simulink library "ammclib_bam_s32k14x"  (Simulink 9.0)
settings: Solver=ode45  StartTime=0.0  StopTime=10.0  RelTol=1e-3
undefined symbols (not defined in the file): f16A1, f16A2, f16B0, f16B1, f16B2, f16C1, f16CC1, f16CC1sc, f16CC1sc_D, f16CC1sc_Q, f16CC1scD, f16CC1scQ, f16CC2, f16CC2sc, f16CC2sc_D, f16CC2sc_Q, f16CC2scD, f16CC2scQ, f16DerivGain, f16EGain, f16FiltCoef, f16HystOff, f16HystOn, f16IGain, f16IntegGain, f16IntegGainFW, f16IntegGainQ, f16Kd, f16Kq, f16Limit, f16LowerLim, f16LowerLimit_D, f16LowerLimit_Q, f16ModIndex, f16OutValOff, f16OutValOn, f16PropGain, f16PropGainFW, f16PropGainQ, f16RampDown, f16RampUp, f16UGain, f16UpperLim, f16UpperLimit, f16UpperLimit_D, f16UpperLimit_Q, f16WIGain, f32A1, f32A2, f32B0, f32B1, f32B2, f32C1, f32CC1, f32CC1sc, f32CC1sc_D, f32CC1sc_Q, f32CC1scD, f32CC1scQ, f32CC2 ... (+122)
(part 3 of 11)

== system ammclib_bam_s32k14x/GMCLIB/bam_f32 ==
  GMCLIB_ClarkInv_F32 : Subsystem  mask(GMCLIB_ClarkInv_F32){}
      mask help: Bit accurate model of inverse Clarke transformation 2ph -> 3ph
      mask init:
      | pos = get_param(gcb, 'Position');width = pos(3) - pos(1); height = pos(4) - pos(2);tX=width/2;tY=height*0.9;
      mask Help: web(fullfile(mbd_s32k_mc_block_help('s32k14x'), 'S32K14XMCLUG.pdf'), '-browser')
      mask Display: color('black');port_label('input',1,'f32Alpha');port_label('input',2,'f32Beta');port_label('output',1,'f32A');port_label('output',2,'f32B');port_label('output',3,'f32C');color('black');disp('GMCLIB_ClarkInv_F32');color('blue');text(tX,tY, 'BAM', 'horizontalAlignment', 'center');
  GMCLIB_Clark_F32 : Subsystem  mask(GMCLIB_Clark_F32){}
      mask help: Bit accurate model of Clarke transformation 3ph -> 2ph.
      mask init:
      | pos = get_param(gcb, 'Position');width = pos(3) - pos(1); height = pos(4) - pos(2);tX=width/2;tY=height*0.9;
      mask Help: web(fullfile(mbd_s32k_mc_block_help('s32k14x'), 'S32K14XMCLUG.pdf'), '-browser')
      mask Display: color('black');port_label('input',1,'f32A');port_label('input',2,'f32B');port_label('input',3,'f32C');port_label('output',1,'f32Alpha');port_label('output',2,'f32Beta');color('black');disp('GMCLIB_Clark_F32');color('blue');text(tX,tY, 'BAM', 'horizontalAlignment', 'center');
  GMCLIB_DecouplingPMSM_F32 : Subsystem  mask(GMCLIB_DecouplingPMSM_F32){f32Kd=f32Kd, s16KdShift=s16KdShift, f32Kq=f32Kq, s16KqShift=s16KqShift}
      mask help: Bit accurate model of decoupling for PMSM model.
      mask init:
      | pos = get_param(gcb, 'Position');width = pos(3) - pos(1); height = pos(4) - pos(2);tX=width/2;tY=height*0.9;
      mask Help: web(fullfile(mbd_s32k_mc_block_help('s32k14x'), 'S32K14XMCLUG.pdf'), '-browser')
      mask Display: color('black');port_label('input',1,'f32Ud');port_label('input',2,'f32Uq');port_label('input',3,'f32Id');port_label('input',4,'f32Iq');port_label('input',5,'f32AngVel');port_label('output',1,'f32UdDec');port_label('output',2,'f32UqDec');color('black');disp('GMCLIB_DecouplingPMSM_F32');color('blue');text(tX,tY, 'BAM', 'horizontalAlignment', 'center');
  GMCLIB_ElimDcBusRip_F32 : Subsystem  mask(GMCLIB_ElimDcBusRip_F32){f32ModIndex=f32ModIndex}
      mask help: Bit accurate model of DC Bus voltage ripple elimination function.
      mask init:
      | pos = get_param(gcb, 'Position');width = pos(3) - pos(1); height = pos(4) - pos(2);tX=width/2;tY=height*0.9;
      mask Help: web(fullfile(mbd_s32k_mc_block_help('s32k14x'), 'S32K14XMCLUG.pdf'), '-browser')
      mask Display: color('black');port_label('input',1,'f32Alpha');port_label('input',2,'f32Beta');port_label('input',3,'f32ArgDcBusMsr');port_label('output',1,'f32AlphaOut');port_label('output',2,'f32BetaOut');color('black');disp('GMCLIB_ElimDcBusRip_F32');color('blue');text(tX,tY, 'BAM', 'horizontalAlignment', 'center');
  GMCLIB_ParkInv_F32 : Subsystem  mask(GMCLIB_ParkInv_F32){}
      mask help: Bit accurate model of Inverse Park transformation 2ph rotational -> 2ph stationary.
      mask init:
      | pos = get_param(gcb, 'Position');width = pos(3) - pos(1); height = pos(4) - pos(2);tX=width/2;tY=height*0.9;
      mask Help: web(fullfile(mbd_s32k_mc_block_help('s32k14x'), 'S32K14XMCLUG.pdf'), '-browser')
      mask Display: color('black');port_label('input',1,'f32D');port_label('input',2,'f32Q');port_label('input',3,'f32Sin');port_label('input',4,'f32Cos');port_label('output',1,'f32Alpha');port_label('output',2,'f32Beta');color('black');disp('GMCLIB_ParkInv_F32');color('blue');text(tX,tY, 'BAM', 'horizontalAlignment', 'center');
  GMCLIB_Park_F32 : Subsystem  mask(GMCLIB_Park_F32){}
      mask help: Bit accurate model of Park transformation 2ph stationary -> 2ph rotational.
      mask init:
      | pos = get_param(gcb, 'Position');width = pos(3) - pos(1); height = pos(4) - pos(2);tX=width/2;tY=height*0.9;
      mask Help: web(fullfile(mbd_s32k_mc_block_help('s32k14x'), 'S32K14XMCLUG.pdf'), '-browser')
      mask Display: color('black');port_label('input',1,'f32Alpha');port_label('input',2,'f32Beta');port_label('input',3,'f32Sin');port_label('input',4,'f32Cos');port_label('output',1,'f32D');port_label('output',2,'f32Q');color('black');disp('GMCLIB_Park_F32');color('blue');text(tX,tY, 'BAM', 'horizontalAlignment', 'center');
  GMCLIB_PwmIct_F32 : Subsystem  mask(GMCLIB_PwmIct_F32){}
      mask help: Bit accurate model of General Sinusoidal PWM.
      mask init:
      | pos = get_param(gcb, 'Position');width = pos(3) - pos(1); height = pos(4) - pos(2);tX=width/2;tY=height*0.9;
      mask Help: web(fullfile(mbd_s32k_mc_block_help('s32k14x'), 'S32K14XMCLUG.pdf'), '-browser')
      mask Display: color('black');port_label('input',1,'f32In1');port_label('input',2,'f32In2');port_label('output',1,'f32Out1');port_label('output',2,'f32Out2');port_label('output',3,'f32Out3');port_label('output',4,'u32Sector');color('black');disp('GMCLIB_PwmIct_F32');color('blue');text(tX,tY, 'BAM', 'horizontalAlignment', 'center');
  GMCLIB_SvmStd_F32 : Subsystem  mask(GMCLIB_SvmStd_F32){}
      mask help: Bit accurate model of Standard Space Vector Modulation.
      mask init:
      | pos = get_param(gcb, 'Position');width = pos(3) - pos(1); height = pos(4) - pos(2);tX=width/2;tY=height*0.9;
      mask Help: web(fullfile(mbd_s32k_mc_block_help('s32k14x'), 'S32K14XMCLUG.pdf'), '-browser')
      mask Display: color('black');port_label('input',1,'f32In1');port_label('input',2,'f32In2');port_label('output',1,'f32Out1');port_label('output',2,'f32Out2');port_label('output',3,'f32Out3');port_label('output',4,'u32Sector');color('black');disp('GMCLIB_SvmStd_F32');color('blue');text(tX,tY, 'BAM', 'horizontalAlignment', 'center');
  GMCLIB_SvmU0n_F32 : Subsystem  mask(GMCLIB_SvmU0n_F32){}
      mask help: Bit accurate model of Standard Space Vector Modulation.
      mask init:
      | pos = get_param(gcb, 'Position');width = pos(3) - pos(1); height = pos(4) - pos(2);tX=width/2;tY=height*0.9;
      mask Help: web(fullfile(mbd_s32k_mc_block_help('s32k14x'), 'S32K14XMCLUG.pdf'), '-browser')
      mask Display: color('black');port_label('input',1,'f32In1');port_label('input',2,'f32In2');port_label('output',1,'f32Out1');port_label('output',2,'f32Out2');port_label('output',3,'f32Out3');port_label('output',4,'u32Sector');color('black');disp('GMCLIB_SvmU0n_F32');color('blue');text(tX,tY, 'BAM', 'horizontalAlignment', 'center');

== system ammclib_bam_s32k14x/GMCLIB/bam_flt ==
  GMCLIB_ClarkInv_FLT : Subsystem  mask(GMCLIB_ClarkInv_FLT){}
      mask help: Bit accurate model of inverse Clarke transformation 2ph -> 3ph
      mask init:
      | pos = get_param(gcb, 'Position');width = pos(3) - pos(1); height = pos(4) - pos(2);tX=width/2;tY=height*0.9;
      mask Help: web(fullfile(mbd_s32k_mc_block_help('s32k14x'), 'S32K14XMCLUG.pdf'), '-browser')
      mask Display: color('black');port_label('input',1,'fltAlpha');port_label('input',2,'fltBeta');port_label('output',1,'fltA');port_label('output',2,'fltB');port_label('output',3,'fltC');color('black');disp('GMCLIB_ClarkInv_FLT');color('blue');text(tX,tY, 'BAM', 'horizontalAlignment', 'center');
  GMCLIB_Clark_FLT : Subsystem  mask(GMCLIB_Clark_FLT){}
      mask help: Bit accurate model of Clarke transformation 3ph -> 2ph.
      mask init:
      | pos = get_param(gcb, 'Position');width = pos(3) - pos(1); height = pos(4) - pos(2);tX=width/2;tY=height*0.9;
      mask Help: web(fullfile(mbd_s32k_mc_block_help('s32k14x'), 'S32K14XMCLUG.pdf'), '-browser')
      mask Display: color('black');port_label('input',1,'fltA');port_label('input',2,'fltB');port_label('input',3,'fltC');port_label('output',1,'fltAlpha');port_label('output',2,'fltBeta');color('black');disp('GMCLIB_Clark_FLT');color('blue');text(tX,tY, 'BAM', 'horizontalAlignment', 'center');
  GMCLIB_DecouplingPMSM_FLT : Subsystem  mask(GMCLIB_DecouplingPMSM_FLT){fltKd=fltKd, fltKq=fltKq}
      mask help: Bit accurate model of decoupling for PMSM model.
      mask init:
      | pos = get_param(gcb, 'Position');width = pos(3) - pos(1); height = pos(4) - pos(2);tX=width/2;tY=height*0.9;
      mask Help: web(fullfile(mbd_s32k_mc_block_help('s32k14x'), 'S32K14XMCLUG.pdf'), '-browser')
      mask Display: color('black');port_label('input',1,'fltUd');port_label('input',2,'fltUq');port_label('input',3,'fltId');port_label('input',4,'fltIq');port_label('input',5,'fltAngVel');port_label('output',1,'fltUdDec');port_label('output',2,'fltUqDec');color('black');disp('GMCLIB_DecouplingPMSM_FLT');color('blue');text(tX,tY, 'BAM', 'horizontalAlignment', 'center');
  GMCLIB_ElimDcBusRip_FLT : Subsystem  mask(GMCLIB_ElimDcBusRip_FLT){fltModIndex=fltModIndex}
      mask help: Bit accurate model of DC Bus voltage ripple elimination function.
      mask init:
      | pos = get_param(gcb, 'Position');width = pos(3) - pos(1); height = pos(4) - pos(2);tX=width/2;tY=height*0.9;
      mask Help: web(fullfile(mbd_s32k_mc_block_help('s32k14x'), 'S32K14XMCLUG.pdf'), '-browser')
      mask Display: color('black');port_label('input',1,'fltAlpha');port_label('input',2,'fltBeta');port_label('input',3,'fltArgDcBusMsr');port_label('output',1,'fltAlphaOut');port_label('output',2,'fltBetaOut');color('black');disp('GMCLIB_ElimDcBusRip_FLT');color('blue');text(tX,tY, 'BAM', 'horizontalAlignment', 'center');
  GMCLIB_ParkInv_FLT : Subsystem  mask(GMCLIB_ParkInv_FLT){}
      mask help: Bit accurate model of Inverse Park transformation 2ph rotational -> 2ph stationary.
      mask init:
      | pos = get_param(gcb, 'Position');width = pos(3) - pos(1); height = pos(4) - pos(2);tX=width/2;tY=height*0.9;
      mask Help: web(fullfile(mbd_s32k_mc_block_help('s32k14x'), 'S32K14XMCLUG.pdf'), '-browser')
      mask Display: color('black');port_label('input',1,'fltD');port_label('input',2,'fltQ');port_label('input',3,'fltSin');port_label('input',4,'fltCos');port_label('output',1,'fltAlpha');port_label('output',2,'fltBeta');color('black');disp('GMCLIB_ParkInv_FLT');color('blue');text(tX,tY, 'BAM', 'horizontalAlignment', 'center');
  GMCLIB_Park_FLT : Subsystem  mask(GMCLIB_Park_FLT){}
      mask help: Bit accurate model of Park transformation 2ph stationary -> 2ph rotational.
      mask init:
      | pos = get_param(gcb, 'Position');width = pos(3) - pos(1); height = pos(4) - pos(2);tX=width/2;tY=height*0.9;
      mask Help: web(fullfile(mbd_s32k_mc_block_help('s32k14x'), 'S32K14XMCLUG.pdf'), '-browser')
      mask Display: color('black');port_label('input',1,'fltAlpha');port_label('input',2,'fltBeta');port_label('input',3,'fltSin');port_label('input',4,'fltCos');port_label('output',1,'fltD');port_label('output',2,'fltQ');color('black');disp('GMCLIB_Park_FLT');color('blue');text(tX,tY, 'BAM', 'horizontalAlignment', 'center');
  GMCLIB_PwmIct_FLT : Subsystem  mask(GMCLIB_PwmIct_FLT){}
      mask help: Bit accurate model of General Sinusoidal PWM.
      mask init:
      | pos = get_param(gcb, 'Position');width = pos(3) - pos(1); height = pos(4) - pos(2);tX=width/2;tY=height*0.9;
      mask Help: web(fullfile(mbd_s32k_mc_block_help('s32k14x'), 'S32K14XMCLUG.pdf'), '-browser')
      mask Display: color('black');port_label('input',1,'fltIn1');port_label('input',2,'fltIn2');port_label('output',1,'fltOut1');port_label('output',2,'fltOut2');port_label('output',3,'fltOut3');port_label('output',4,'u32Sector');color('black');disp('GMCLIB_PwmIct_FLT');color('blue');text(tX,tY, 'BAM', 'horizontalAlignment', 'center');
  GMCLIB_SvmStd_FLT : Subsystem  mask(GMCLIB_SvmStd_FLT){}
      mask help: Bit accurate model of Standard Space Vector Modulation.
      mask init:
      | pos = get_param(gcb, 'Position');width = pos(3) - pos(1); height = pos(4) - pos(2);tX=width/2;tY=height*0.9;
      mask Help: web(fullfile(mbd_s32k_mc_block_help('s32k14x'), 'S32K14XMCLUG.pdf'), '-browser')
      mask Display: color('black');port_label('input',1,'fltIn1');port_label('input',2,'fltIn2');port_label('output',1,'fltOut1');port_label('output',2,'fltOut2');port_label('output',3,'fltOut3');port_label('output',4,'u32Sector');color('black');disp('GMCLIB_SvmStd_FLT');color('blue');text(tX,tY, 'BAM', 'horizontalAlignment', 'center');
  GMCLIB_SvmU0n_FLT : Subsystem  mask(GMCLIB_SvmU0n_FLT){}
      mask help: Bit accurate model of Standard Space Vector Modulation.
      mask init:
      | pos = get_param(gcb, 'Position');width = pos(3) - pos(1); height = pos(4) - pos(2);tX=width/2;tY=height*0.9;
      mask Help: web(fullfile(mbd_s32k_mc_block_help('s32k14x'), 'S32K14XMCLUG.pdf'), '-browser')
      mask Display: color('black');port_label('input',1,'fltIn1');port_label('input',2,'fltIn2');port_label('output',1,'fltOut1');port_label('output',2,'fltOut2');port_label('output',3,'fltOut3');port_label('output',4,'u32Sector');color('black');disp('GMCLIB_SvmU0n_FLT');color('blue');text(tX,tY, 'BAM', 'horizontalAlignment', 'center');

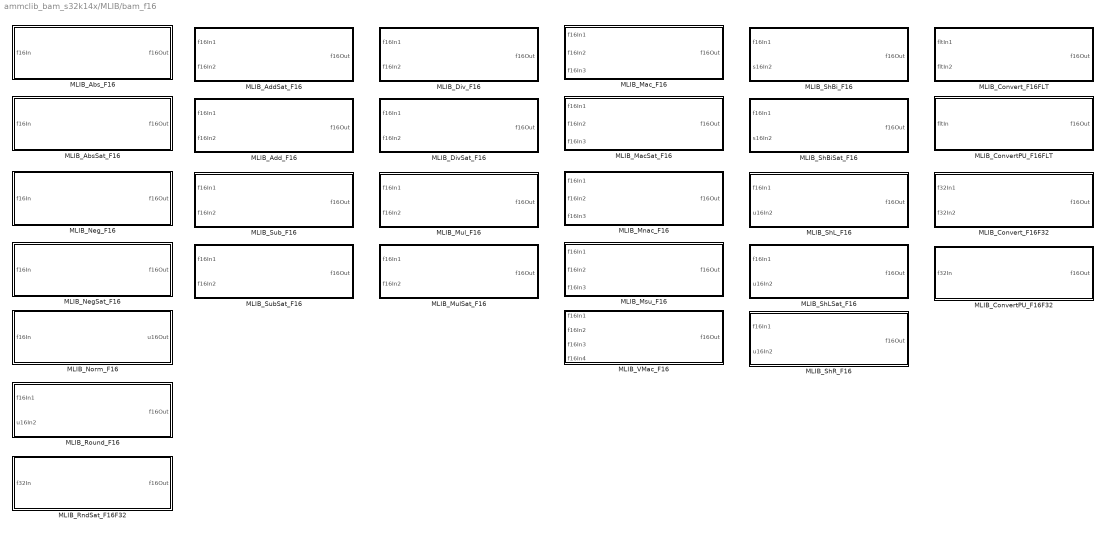
== system ammclib_bam_s32k14x/MLIB/bam_f16 ==
  MLIB_AbsSat_F16 : Subsystem  mask(MLIB_AbsSat_F16){}
      mask help: Bit accurate model for absolute value of input value. The output is saturated if necessary. All parameters as well as input and output are 16bit integers.
      mask init:
      | pos = get_param(gcb, 'Position');width = pos(3) - pos(1); height = pos(4) - pos(2);tX=width/2;tY=height*0.9;
      mask Help: web(fullfile(mbd_s32k_mc_block_help('s32k14x'), 'S32K14XMCLUG.pdf'), '-browser')
      mask Display: color('black');port_label('input',1,'f16In');port_label('output',1,'f16Out');color('black');disp('MLIB_AbsSat_F16');color('blue');text(tX,tY, 'BAM', 'horizontalAlignment', 'center');
  MLIB_Abs_F16 : Subsystem  mask(MLIB_Abs_F16){}
      mask help: Bit accurate model for absolute value of input value. All parameters as well as input and output are 16bit integers.
      mask init:
      | pos = get_param(gcb, 'Position');width = pos(3) - pos(1); height = pos(4) - pos(2);tX=width/2;tY=height*0.9;
      mask Help: web(fullfile(mbd_s32k_mc_block_help('s32k14x'), 'S32K14XMCLUG.pdf'), '-browser')
      mask Display: color('black');port_label('input',1,'f16In');port_label('output',1,'f16Out');color('black');disp('MLIB_Abs_F16');color('blue');text(tX,tY, 'BAM', 'horizontalAlignment', 'center');
  MLIB_AddSat_F16 : Subsystem  mask(MLIB_AddSat_F16){}
      mask help: Bit accurate model of saturated sum of two input values. All parameters as well as input and output are 16bit integers.
      mask init:
      | pos = get_param(gcb, 'Position');width = pos(3) - pos(1); height = pos(4) - pos(2);tX=width/2;tY=height*0.9;
      mask Help: web(fullfile(mbd_s32k_mc_block_help('s32k14x'), 'S32K14XMCLUG.pdf'), '-browser')
      mask Display: color('black');port_label('input',1,'f16In1');port_label('input',2,'f16In2');port_label('output',1,'f16Out');color('black');disp('MLIB_AddSat_F16');color('blue');text(tX,tY, 'BAM', 'horizontalAlignment', 'center');
  MLIB_Add_F16 : Subsystem  mask(MLIB_Add_F16){}
      mask help: Bit accurate model of sum of two input values. All parameters as well as input and output are 16bit integers.
      mask init:
      | pos = get_param(gcb, 'Position');width = pos(3) - pos(1); height = pos(4) - pos(2);tX=width/2;tY=height*0.9;
      mask Help: web(fullfile(mbd_s32k_mc_block_help('s32k14x'), 'S32K14XMCLUG.pdf'), '-browser')
      mask Display: color('black');port_label('input',1,'f16In1');port_label('input',2,'f16In2');port_label('output',1,'f16Out');color('black');disp('MLIB_Add_F16');color('blue');text(tX,tY, 'BAM', 'horizontalAlignment', 'center');
  MLIB_ConvertPU_F16F32 : Subsystem  mask(MLIB_ConvertPU_F16){}
      mask help: Bit accurate model for conversion value of input value. Input parameter is considered as 32-bit integer and output value is considered as 16-bit integer value.
      mask init:
      | pos = get_param(gcb, 'Position');width = pos(3) - pos(1); height = pos(4) - pos(2);tX=width/2;tY=height*0.9;
      mask Help: web(fullfile(mbd_s32k_mc_block_help('s32k14x'), 'S32K14XMCLUG.pdf'), '-browser')
      mask Display: color('black');port_label('input',1,'f32In');port_label('output',1,'f16Out');color('black');disp('MLIB_ConvertPU_F16F32');color('blue');text(tX,tY, 'BAM', 'horizontalAlignment', 'center');
  MLIB_ConvertPU_F16FLT : Subsystem  mask(MLIB_ConvertPU_F16){}
      mask help: Bit accurate model for conversion value of input value. Input parameter is considered as single precision floating point value and output value is considered as 16-bit integer value.
      mask init:
      | pos = get_param(gcb, 'Position');width = pos(3) - pos(1); height = pos(4) - pos(2);tX=width/2;tY=height*0.9;
      mask Help: web(fullfile(mbd_s32k_mc_block_help('s32k14x'), 'S32K14XMCLUG.pdf'), '-browser')
      mask Display: color('black');port_label('input',1,'fltIn');port_label('output',1,'f16Out');color('black');disp('MLIB_ConvertPU_F16FLT');color('blue');text(tX,tY, 'BAM', 'horizontalAlignment', 'center');
  MLIB_Convert_F16F32 : Subsystem  mask(MLIB_Convert_F16F32){}
      mask help: Bit accurate model for conversion value of input value. Input parameter is considered as 32-bit integer and output value is considered as 16-bit integer value.
      mask init:
      | pos = get_param(gcb, 'Position');width = pos(3) - pos(1); height = pos(4) - pos(2);tX=width/2;tY=height*0.9;
      mask Help: web(fullfile(mbd_s32k_mc_block_help('s32k14x'), 'S32K14XMCLUG.pdf'), '-browser')
      mask Display: color('black');port_label('input',1,'f32In1');port_label('input',2,'f32In2');port_label('output',1,'f16Out');color('black');disp('MLIB_Convert_F16F32');color('blue');text(tX,tY, 'BAM', 'horizontalAlignment', 'center');
  MLIB_Convert_F16FLT : Subsystem  mask(MLIB_Convert_F16FLT){}
      mask help: Bit accurate model for conversion value of input value. Input parameter is considered as single precision floating point value and output value is considered as 16-bit integer value.
      mask init:
      | pos = get_param(gcb, 'Position');width = pos(3) - pos(1); height = pos(4) - pos(2);tX=width/2;tY=height*0.9;
      mask Help: web(fullfile(mbd_s32k_mc_block_help('s32k14x'), 'S32K14XMCLUG.pdf'), '-browser')
      mask Display: color('black');port_label('input',1,'fltIn1');port_label('input',2,'fltIn2');port_label('output',1,'f16Out');color('black');disp('MLIB_Convert_F16FLT');color('blue');text(tX,tY, 'BAM', 'horizontalAlignment', 'center');
  MLIB_DivSat_F16 : Subsystem  mask(MLIB_DivSat_F16){}
      mask help: Bit accurate model of multiplication of two input values. All parameters as well as input and output are 16bit integers.
      mask init:
      | pos = get_param(gcb, 'Position');width = pos(3) - pos(1); height = pos(4) - pos(2);tX=width/2;tY=height*0.9;
      mask Help: web(fullfile(mbd_s32k_mc_block_help('s32k14x'), 'S32K14XMCLUG.pdf'), '-browser')
      mask Display: color('black');port_label('input',1,'f16In1');port_label('input',2,'f16In2');port_label('output',1,'f16Out');color('black');disp('MLIB_DivSat_F16');color('blue');text(tX,tY, 'BAM', 'horizontalAlignment', 'center');
  MLIB_Div_F16 : Subsystem  mask(MLIB_Div_F16){}
      mask help: Bit accurate model of multiplication of two input values. All parameters as well as input and output are 16bit integers.
      mask init:
      | pos = get_param(gcb, 'Position');width = pos(3) - pos(1); height = pos(4) - pos(2);tX=width/2;tY=height*0.9;
      mask Help: web(fullfile(mbd_s32k_mc_block_help('s32k14x'), 'S32K14XMCLUG.pdf'), '-browser')
      mask Display: color('black');port_label('input',1,'f16In1');port_label('input',2,'f16In2');port_label('output',1,'f16Out');color('black');disp('MLIB_Div_F16');color('blue');text(tX,tY, 'BAM', 'horizontalAlignment', 'center');
  MLIB_MacSat_F16 : Subsystem  mask(MLIB_MacSat_F16){}
      mask help: Bit accurate model of saturated multiply-accumulate of input values, staturated if necessary. All parameters as well as input and output are 16bit integers.
      mask init:
      | pos = get_param(gcb, 'Position');width = pos(3) - pos(1); height = pos(4) - pos(2);tX=width/2;tY=height*0.9;
      mask Help: web(fullfile(mbd_s32k_mc_block_help('s32k14x'), 'S32K14XMCLUG.pdf'), '-browser')
      mask Display: color('black');port_label('input',1,'f16In1');port_label('input',2,'f16In2');port_label('input',3,'f16In3');port_label('output',1,'f16Out');color('black');disp('MLIB_MacSat_F16');color('blue');text(tX,tY, 'BAM', 'horizontalAlignment', 'center');
  MLIB_Mac_F16 : Subsystem  mask(MLIB_Mac_F16){}
      mask help: Bit accurate model of multiply accumulate function. All parameters as well as input and output are 16bit integers.
      mask init:
      | pos = get_param(gcb, 'Position');width = pos(3) - pos(1); height = pos(4) - pos(2);tX=width/2;tY=height*0.9;
      mask Help: web(fullfile(mbd_s32k_mc_block_help('s32k14x'), 'S32K14XMCLUG.pdf'), '-browser')
      mask Display: color('black');port_label('input',1,'f16In1');port_label('input',2,'f16In2');port_label('input',3,'f16In3');port_label('output',1,'f16Out');color('black');disp('MLIB_Mac_F16');color('blue');text(tX,tY, 'BAM', 'horizontalAlignment', 'center');
  MLIB_Mnac_F16 : Subsystem  mask(MLIB_Mnac_F16){}
      mask help: Bit accurate model of multiply-negative-accumulate function. All parameters as well as input and output are 16bit integers.
      mask init:
      | pos = get_param(gcb, 'Position');width = pos(3) - pos(1); height = pos(4) - pos(2);tX=width/2;tY=height*0.9;
      mask Help: web(fullfile(mbd_s32k_mc_block_help('s32k14x'), 'S32K14XMCLUG.pdf'), '-browser')
      mask Display: color('black');port_label('input',1,'f16In1');port_label('input',2,'f16In2');port_label('input',3,'f16In3');port_label('output',1,'f16Out');color('black');disp('MLIB_Mnac_F16');color('blue');text(tX,tY, 'BAM', 'horizontalAlignment', 'center');
  MLIB_Msu_F16 : Subsystem  mask(MLIB_Msu_F16){}
      mask help: Bit accurate model of multiply-subtract-from function. All parameters as well as input and output are 16bit integers.
      mask init:
      | pos = get_param(gcb, 'Position');width = pos(3) - pos(1); height = pos(4) - pos(2);tX=width/2;tY=height*0.9;
      mask Help: web(fullfile(mbd_s32k_mc_block_help('s32k14x'), 'S32K14XMCLUG.pdf'), '-browser')
      mask Display: color('black');port_label('input',1,'f16In1');port_label('input',2,'f16In2');port_label('input',3,'f16In3');port_label('output',1,'f16Out');color('black');disp('MLIB_Msu_F16');color('blue');text(tX,tY, 'BAM', 'horizontalAlignment', 'center');
  MLIB_MulSat_F16 : Subsystem  mask(MLIB_MulSat_F16){}
      mask help: Bit accurate model of saturated multiplication of two input values. All parameters as well as input and output are 16bit integers.
      mask init:
      | pos = get_param(gcb, 'Position');width = pos(3) - pos(1); height = pos(4) - pos(2);tX=width/2;tY=height*0.9;
      mask Help: web(fullfile(mbd_s32k_mc_block_help('s32k14x'), 'S32K14XMCLUG.pdf'), '-browser')
      mask Display: color('black');port_label('input',1,'f16In1');port_label('input',2,'f16In2');port_label('output',1,'f16Out');color('black');disp('MLIB_MulSat_F16');color('blue');text(tX,tY, 'BAM', 'horizontalAlignment', 'center');
  MLIB_Mul_F16 : Subsystem  mask(MLIB_Mul_F16){}
      mask help: Bit accurate model of multiplication of two input values. All parameters as well as input and output are 16bit integers.
      mask init:
      | pos = get_param(gcb, 'Position');width = pos(3) - pos(1); height = pos(4) - pos(2);tX=width/2;tY=height*0.9;
      mask Help: web(fullfile(mbd_s32k_mc_block_help('s32k14x'), 'S32K14XMCLUG.pdf'), '-browser')
      mask Display: color('black');port_label('input',1,'f16In1');port_label('input',2,'f16In2');port_label('output',1,'f16Out');color('black');disp('MLIB_Mul_F16');color('blue');text(tX,tY, 'BAM', 'horizontalAlignment', 'center');
  MLIB_NegSat_F16 : Subsystem  mask(MLIB_NegSat_F16){}
      mask help: Bit accurate model for negative value of input value. The output is saturated if necessary. All parameters as well as input and output are 16bit integers.
      mask init:
      | pos = get_param(gcb, 'Position');width = pos(3) - pos(1); height = pos(4) - pos(2);tX=width/2;tY=height*0.9;
      mask Help: web(fullfile(mbd_s32k_mc_block_help('s32k14x'), 'S32K14XMCLUG.pdf'), '-browser')
      mask Display: color('black');port_label('input',1,'f16In');port_label('output',1,'f16Out');color('black');disp('MLIB_NegSat_F16');color('blue');text(tX,tY, 'BAM', 'horizontalAlignment', 'center');
  MLIB_Neg_F16 : Subsystem  mask(MLIB_Neg_F16){}
      mask help: Bit accurate model for negative value of input value. All parameters as well as input and output are 16bit integers.
      mask init:
      | pos = get_param(gcb, 'Position');width = pos(3) - pos(1); height = pos(4) - pos(2);tX=width/2;tY=height*0.9;
      mask Help: web(fullfile(mbd_s32k_mc_block_help('s32k14x'), 'S32K14XMCLUG.pdf'), '-browser')
      mask Display: color('black');port_label('input',1,'f16In');port_label('output',1,'f16Out');color('black');disp('MLIB_Neg_F16');color('blue');text(tX,tY, 'BAM', 'horizontalAlignment', 'center');
  MLIB_Norm_F16 : Subsystem  mask(MLIB_Norm_F16){}
      mask help: Bit accurate model of the normalization function. The function counts the number of left shift needed for normalization of the input fractional value.
      mask init:
      | pos = get_param(gcb, 'Position');width = pos(3) - pos(1); height = pos(4) - pos(2);tX=width/2;tY=height*0.9;
      mask Help: web(fullfile(mbd_s32k_mc_block_help('s32k14x'), 'S32K14XMCLUG.pdf'), '-browser')
      mask Display: color('black');port_label('input',1,'f16In');port_label('output',1,'u16Out');color('black');disp('MLIB_Norm_F16');color('blue');text(tX,tY, 'BAM', 'horizontalAlignment', 'center');
  MLIB_RndSat_F16F32 : Subsystem  mask(MLIB_RndSat_F16F32){}
      mask help: Bit accurate model for conversion of input value. Input parameter is considered as 32-bit integer and output value is considered as 16-bit integer value.
      mask init:
      | pos = get_param(gcb, 'Position');width = pos(3) - pos(1); height = pos(4) - pos(2);tX=width/2;tY=height*0.9;
      mask Help: web(fullfile(mbd_s32k_mc_block_help('s32k14x'), 'S32K14XMCLUG.pdf'), '-browser')
      mask Display: color('black');port_label('input',1,'f32In');port_label('output',1,'f16Out');color('black');disp('MLIB_RndSat_F16F32');color('blue');text(tX,tY, 'BAM', 'horizontalAlignment', 'center');
  MLIB_Round_F16 : Subsystem  mask(MLIB_Round_F16){}
      mask help: Bit accurate model of the fuction rounds the first input value for number of digits defined by second parameter and saturate automaticaly. All parameters as well as input and output are 16bit integers.
      mask init:
      | pos = get_param(gcb, 'Position');width = pos(3) - pos(1); height = pos(4) - pos(2);tX=width/2;tY=height*0.9;
      mask Help: web(fullfile(mbd_s32k_mc_block_help('s32k14x'), 'S32K14XMCLUG.pdf'), '-browser')
      mask Display: color('black');port_label('input',1,'f16In1');port_label('input',2,'u16In2');port_label('output',1,'f16Out');color('black');disp('MLIB_Round_F16');color('blue');text(tX,tY, 'BAM', 'horizontalAlignment', 'center');
  MLIB_ShBiSat_F16 : Subsystem  mask(MLIB_ShBiSat_F16){}
      mask help: Bit accurate model of the fuction shifts the first parameter to left or right by number defined by second parameter and saturate if necessary. If the sign of second parameter is negative, shift to right. All parameters as well as input and output are 16bit integers.
      mask init:
      | pos = get_param(gcb, 'Position');width = pos(3) - pos(1); height = pos(4) - pos(2);tX=width/2;tY=height*0.9;
      mask Help: web(fullfile(mbd_s32k_mc_block_help('s32k14x'), 'S32K14XMCLUG.pdf'), '-browser')
      mask Display: color('black');port_label('input',1,'f16In1');port_label('input',2,'s16In2');port_label('output',1,'f16Out');color('black');disp('MLIB_ShBiSat_F16');color('blue');text(tX,tY, 'BAM', 'horizontalAlignment', 'center');
  MLIB_ShBi_F16 : Subsystem  mask(MLIB_ShBi_F16){}
      mask help: Bit accurate model of the fuction shifts the first parameter to left or right by number defined by second parameter. If the sign of second parameter is negative, shift to right. All parameters as well as input and output are 16bit integers.
      mask init:
      | pos = get_param(gcb, 'Position');width = pos(3) - pos(1); height = pos(4) - pos(2);tX=width/2;tY=height*0.9;
      mask Help: web(fullfile(mbd_s32k_mc_block_help('s32k14x'), 'S32K14XMCLUG.pdf'), '-browser')
      mask Display: color('black');port_label('input',1,'f16In1');port_label('input',2,'s16In2');port_label('output',1,'f16Out');color('black');disp('MLIB_ShBi_F16');color('blue');text(tX,tY, 'BAM', 'horizontalAlignment', 'center');
  MLIB_ShLSat_F16 : Subsystem  mask(MLIB_ShLSat_F16){}
      mask help: Bit accurate model of the fuction shifts the first parameter to left by number defined by second parameter and saturate if necessary. All parameters as well as input and output are 16bit integers.
      mask init:
      | pos = get_param(gcb, 'Position');width = pos(3) - pos(1); height = pos(4) - pos(2);tX=width/2;tY=height*0.9;
      mask Help: web(fullfile(mbd_s32k_mc_block_help('s32k14x'), 'S32K14XMCLUG.pdf'), '-browser')
      mask Display: color('black');port_label('input',1,'f16In1');port_label('input',2,'u16In2');port_label('output',1,'f16Out');color('black');disp('MLIB_ShLSat_F16');color('blue');text(tX,tY, 'BAM', 'horizontalAlignment', 'center');
  MLIB_ShL_F16 : Subsystem  mask(MLIB_ShL_F16){}
      mask help: Bit accurate model of the fuction shifts the first parameter to left by number defined by second parameter. All parameters as well as input and output are 16bit integers.
      mask init:
      | pos = get_param(gcb, 'Position');width = pos(3) - pos(1); height = pos(4) - pos(2);tX=width/2;tY=height*0.9;
      mask Help: web(fullfile(mbd_s32k_mc_block_help('s32k14x'), 'S32K14XMCLUG.pdf'), '-browser')
      mask Display: color('black');port_label('input',1,'f16In1');port_label('input',2,'u16In2');port_label('output',1,'f16Out');color('black');disp('MLIB_ShL_F16');color('blue');text(tX,tY, 'BAM', 'horizontalAlignment', 'center');
  MLIB_ShR_F16 : Subsystem  mask(MLIB_ShR_F16){}
      mask help: Bit accurate model of the fuction shifts the first parameter to right by number defined by second parameter. All parameters as well as input and output are 16bit integers.
      mask init:
      | pos = get_param(gcb, 'Position');width = pos(3) - pos(1); height = pos(4) - pos(2);tX=width/2;tY=height*0.9;
      mask Help: web(fullfile(mbd_s32k_mc_block_help('s32k14x'), 'S32K14XMCLUG.pdf'), '-browser')
      mask Display: color('black');port_label('input',1,'f16In1');port_label('input',2,'u16In2');port_label('output',1,'f16Out');color('black');disp('MLIB_ShR_F16');color('blue');text(tX,tY, 'BAM', 'horizontalAlignment', 'center');
  MLIB_SubSat_F16 : Subsystem  mask(MLIB_SubSat_F16){}
      mask help: Bit accurate model of saturated subtraction of two input values. All parameters as well as input and output are 16bit integers.
      mask init:
      | pos = get_param(gcb, 'Position');width = pos(3) - pos(1); height = pos(4) - pos(2);tX=width/2;tY=height*0.9;
      mask Help: web(fullfile(mbd_s32k_mc_block_help('s32k14x'), 'S32K14XMCLUG.pdf'), '-browser')
      mask Display: color('black');port_label('input',1,'f16In1');port_label('input',2,'f16In2');port_label('output',1,'f16Out');color('black');disp('MLIB_SubSat_F16');color('blue');text(tX,tY, 'BAM', 'horizontalAlignment', 'center');
  MLIB_Sub_F16 : Subsystem  mask(MLIB_Sub_F16){}
      mask help: Bit accurate model of subtract of two input values. All parameters as well as input and output are 16bit integers.
      mask init:
      | pos = get_param(gcb, 'Position');width = pos(3) - pos(1); height = pos(4) - pos(2);tX=width/2;tY=height*0.9;
      mask Help: web(fullfile(mbd_s32k_mc_block_help('s32k14x'), 'S32K14XMCLUG.pdf'), '-browser')
      mask Display: color('black');port_label('input',1,'f16In1');port_label('input',2,'f16In2');port_label('output',1,'f16Out');color('black');disp('MLIB_Sub_F16');color('blue');text(tX,tY, 'BAM', 'horizontalAlignment', 'center');
  MLIB_VMac_F16 : Subsystem  mask(MLIB_VMac_F16){}
      mask help: Bit accurate model of vector multiply accumulate function. All parameters as well as input and output are 16-bit integers.
      mask init:
      | pos = get_param(gcb, 'Position');width = pos(3) - pos(1); height = pos(4) - pos(2);tX=width/2;tY=height*0.9;
      mask Help: web(fullfile(mbd_s32k_mc_block_help('s32k14x'), 'S32K14XMCLUG.pdf'), '-browser')
      mask Display: color('black');port_label('input',1,'f16In1');port_label('input',2,'f16In2');port_label('input',3,'f16In3');port_label('input',4,'f16In4');port_label('output',1,'f16Out');color('black');disp('MLIB_VMac_F16');color('blue');text(tX,tY, 'BAM', 'horizontalAlignment', 'center');
